simulink model "LQR_controller"  (R2017a)
settings: Solver=VariableStepAuto  StartTime=0.0  StopTime=20  RelTol=1e-3  EnableMultiTasking=on
model workspace (MAT data in the model file):
  M = 1000
  X0 = 0.174532925199
  l1 = 20
  l2 = 10
  m1 = 100
  m2 = 100
undefined symbols (not defined in the file): K
settings Model: Creator=Rishabh  LastModifiedBy=manas
settings OptimizationCC: LifeSpan=inf
settings DebuggingCC: SFUnexpectedBacktrackingDiag=warning  SFNoUnconditionalDefaultTransitionDiag=warning  SFExecutionAtInitializationDiag=none
settings GRTTargetCC: TargetLangStandard=C89/C90 (ANSI)  GeneratePreprocessorConditionals=Disable all
settings ConfigComp: CovMetricSettings=dw  CovHtmlReporting=on  CovSaveCumulativeToWorkspaceVar=on  CovSaveSingleToWorkspaceVar=on  CovExternalEMLEnable=off

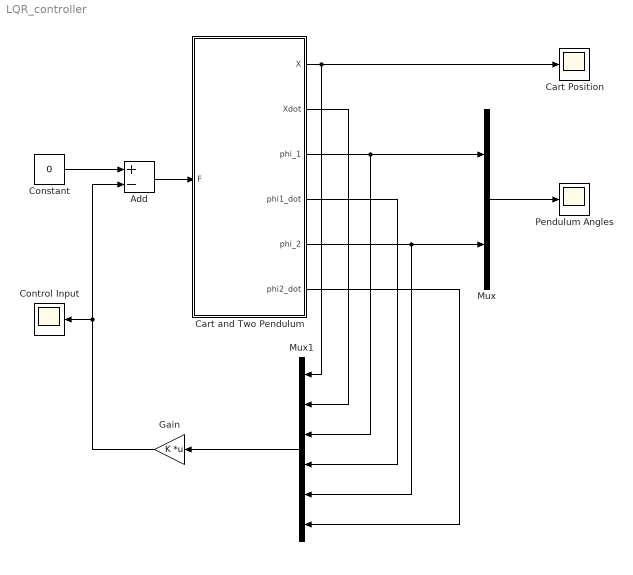
== system LQR_controller ==
  Add : Sum  Inputs=+-
  Cart Position : Scope
  "Cart and Two Pendulum " : Subsystem
  Constant : Constant  Value=0
  Control Input : Scope
  Gain : Gain  Gain=K  Multiplication=Matrix(K*u)
  Mux : Mux  Inputs=2
  Mux1 : Mux  Inputs=6
  Pendulum Angles : Scope
  wires:
  "Cart and Two Pendulum "/1(X) -> Mux1/1, Cart Position/1
  "Cart and Two Pendulum "/3(phi_1) -> Mux1/3, Mux/1
  Mux/1 -> Pendulum Angles/1
  Constant/1 -> Add/1
  Add/1 -> "Cart and Two Pendulum "/1(F)
  "Cart and Two Pendulum "/5(phi_2) -> Mux1/5, Mux/2
  "Cart and Two Pendulum "/2(Xdot) -> Mux1/2
  "Cart and Two Pendulum "/4(phi1_dot) -> Mux1/4
  "Cart and Two Pendulum "/6(phi2_dot) -> Mux1/6
  Mux1/1 -> Gain/1
  Gain/1 -> Control Input/1, Add/2

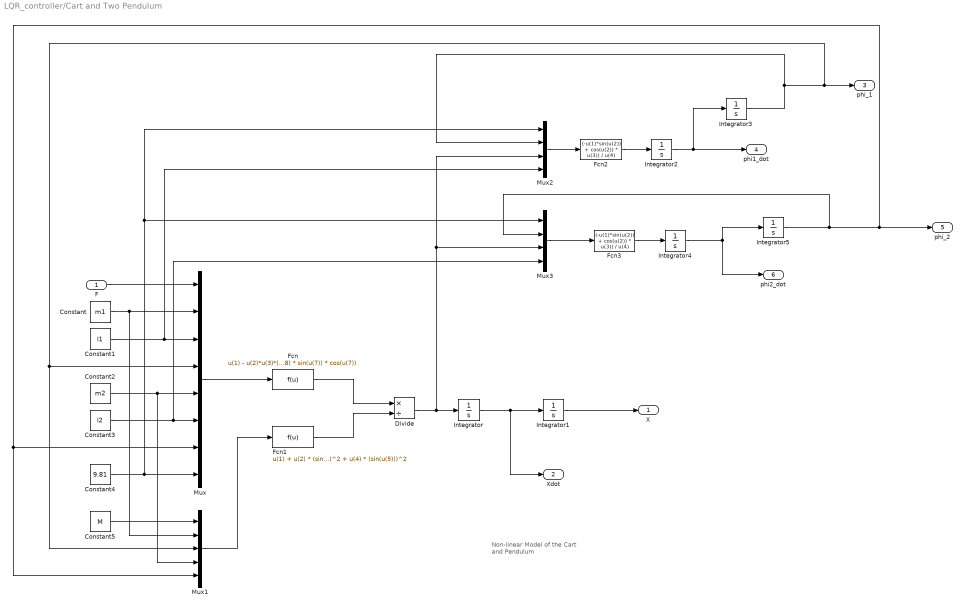
== system LQR_controller/Cart and Two Pendulum  ==
  note: Non-linear Model of the Cart and Pendulum
  F : Inport
  Constant : Constant  Value=m1
  Constant1 : Constant  Value=l1
  Constant2 : Constant  Value=m2
  Constant3 : Constant  Value=l2
  Constant4 : Constant  Value=9.81
  Constant5 : Constant  Value=M
  Divide : Product  Inputs=*/
  Fcn : Fcn  Expr=u(1) - u(2)*u(3)*(u(4)^2)*sin(u(4)) - u(5) * u(6) * (u(7)^2)*sin(u(7))-u(2)*u(8)*sin(u(4))*cos(u(4)) - u(5) * u(8) * sin(u(7)) * cos(u(7))
  Fcn1 : Fcn  Expr=u(1) + u(2) * (sin(u(3)))^2 + u(4) * (sin(u(5)))^2
  Fcn2 : Fcn  Expr=(-u(1)*sin(u(2)) + cos(u(2)) * u(3)) / u(4)
  Fcn3 : Fcn  Expr=(-u(1)*sin(u(2)) + cos(u(2)) * u(3)) / u(4)
  Integrator{,1..2,4} (4 alike) : Integrator
  Integrator3 : Integrator  InitialCondition=10*pi/180
  Integrator5 : Integrator  InitialCondition=15*pi/180
  Mux : Mux  Inputs=8
  Mux1 : Mux  Inputs=5
  Mux2 : Mux
  Mux3 : Mux
  X : Outport
  Xdot : Outport  Port=2
  phi_1 : Outport  Port=3
  phi1_dot : Outport  Port=4
  phi_2 : Outport  Port=5
  phi2_dot : Outport  Port=6
  wires:
  Mux1/1 -> Fcn1/1
  Mux3/1 -> Fcn3/1
  Fcn/1 -> Divide/1
  Integrator2/1 -> phi1_dot/1, Integrator3/1
  Integrator4/1 -> Integrator5/1, phi2_dot/1
  Integrator5/1 -> phi_2/1, Mux1/5, Mux/7, Mux3/2
  Integrator3/1 -> phi_1/1, Mux1/3, Mux/4, Mux2/2
  Divide/1 -> Mux2/3, Mux3/3, Integrator/1
  Constant5/1 -> Mux1/1
  Constant3/1 -> Mux3/4, Mux/6
  Constant2/1 -> Mux1/4, Mux/5
  Constant/1 -> Mux1/2, Mux/2
  F/1 -> Mux/1
  Constant1/1 -> Mux2/4, Mux/3
  Integrator/1 -> Xdot/1, Integrator1/1
  Fcn2/1 -> Integrator2/1
  Constant4/1 -> Mux2/1, Mux3/1, Mux/8
  Mux2/1 -> Fcn2/1
  Integrator1/1 -> X/1
  Mux/1 -> Fcn/1
  Fcn3/1 -> Integrator4/1
  Fcn1/1 -> Divide/2
